simulink model "supervisoryController_ref"  (R2019b)
settings: Solver=FixedStepDiscrete  StartTime=0.0  StopTime=10  FixedStep=0.01  RelTol=1e-3  EnableMultiTasking=on
PreLoadFcn:
  | Ts1 = 0.01;
  | Ts2 = 0.1;
InitFcn:
  | initACCParams_pid;
model workspace (MAT data in the model file):
  firstWarning = 1
  originalScenarioChecksum = '3C3E23DDE530CB8BEC76DD6DBB66960A'
undefined symbols (not defined in the file): default_spacing, DiscIntNeverNeededParam, time_gap
libraries: simulink x1
settings Model: EnablePacing=on  Creator=sseshadr  LastModifiedBy=cdsouza
settings SolverCC: AutoInsertRateTranBlk=on
settings DataIOCC: SaveOutput=off  SaveTime=off
settings OptimizationCC: GainParamInheritBuiltInType=on  UseFloatMulNetSlope=on  EnableMemcpy=off  PassReuseOutputArgsAs=Individual arguments  ZeroExternalMemoryAtStartup=off  ZeroInternalMemoryAtStartup=off  NoFixptDivByZeroProtection=on  EfficientFloat2IntCast=on  LifeSpan=1  OptimizeBlockOrder=speed  DifferentSizesBufferReuse=on  EfficientTunableParamExpr=on
settings DebuggingCC: ParameterTunabilityLossMsg=error
settings HardwareCC: ProdLongLongMode=on
settings SFSimCC: MATLABDynamicMemAlloc=off
settings RTWCC: SystemTargetFile=ert.tlc  TemplateMakefile=ert_default_tmf  GenerateReport=on  IncludeHyperlinkInReport=on  LaunchReport=on  GenerateTraceInfo=on  GenerateTraceReport=on  GenerateTraceReportSl=on  GenerateTraceReportSf=on  GenerateTraceReportEml=on  GenerateCodeMetricsReport=on
settings CodeAppCC: ForceParamTrailComments=on  IgnoreCustomStorageClasses=off  OperatorAnnotations=on  SimulinkDataObjDesc=on  SFDataObjDesc=on  CustomSymbolStrGlobalVar=rt$N$M  CustomSymbolStrType=$N$M  CustomSymbolStrFcn=$N$M$F  CustomSymbolStrMacro=$N$M  InsertBlockDesc=on
settings ERTTargetCC: TargetLangStandard=C99 (ISO)  GenerateSampleERTMain=on  IncludeMdlTerminateFcn=off  CombineSignalStateStructs=on  SupportAbsoluteTime=off  SupportComplex=off  SupportNonInlinedSFcns=on  ERTCustomFileTemplate=example_file_process.tlc

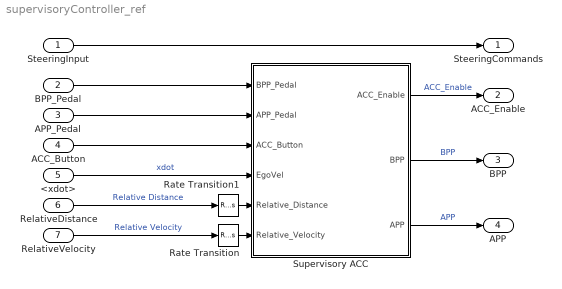
== system supervisoryController_ref ==
  "SteeringInput " : Inport  OutDataTypeStr=double  PortDimensions=1  SampleTime=Ts1
  BPP_Pedal : Inport  Port=2  OutDataTypeStr=double  PortDimensions=1  SampleTime=Ts1
  APP_Pedal : Inport  Port=3  OutDataTypeStr=double  PortDimensions=1  SampleTime=Ts1
  ACC_Button : Inport  Port=4  OutDataTypeStr=double  PortDimensions=1  SampleTime=Ts1
  <xdot> : Inport  Port=5  OutDataTypeStr=double  PortDimensions=1  SampleTime=Ts1
  RelativeDistance : Inport  Port=6  OutDataTypeStr=double  PortDimensions=[1 1]  SampleTime=Ts2
  RelativeVelocity : Inport  Port=7  OutDataTypeStr=double  PortDimensions=[1 1]  SampleTime=Ts2
  Rate Transition : RateTransition
  Rate Transition1 : RateTransition
  Supervisory ACC : Stateflow chart  BlockKeywords=__PRM__SERIALIZED__DATA__:Stateflow Chart,Stateflow Diagram  TreatAsAtomicUnit=on
  SteeringCommands : Outport  OutDataTypeStr=double  PortDimensions=1
  ACC_Enable : Outport  Port=2  OutDataTypeStr=double  PortDimensions=1
  BPP : Outport  Port=3  OutDataTypeStr=double  PortDimensions=1
  APP : Outport  Port=4  OutDataTypeStr=double  PortDimensions=1
  wires:
  BPP_Pedal/1 -> Supervisory ACC/1(BPP_Pedal)
  Supervisory ACC/2(BPP) -> BPP/1  "BPP"
  Supervisory ACC/3(APP) -> APP/1  "APP"
  Supervisory ACC/1(ACC_Enable) -> ACC_Enable/1  "ACC_Enable"
  RelativeDistance/1 -> Rate Transition1/1  "Relative Distance"
  ACC_Button/1 -> Supervisory ACC/3(ACC_Button)
  <xdot>/1 -> Supervisory ACC/4(EgoVel)  "xdot"
  APP_Pedal/1 -> Supervisory ACC/2(APP_Pedal)
  "SteeringInput "/1 -> SteeringCommands/1
  RelativeVelocity/1 -> Rate Transition/1  "Relative Velocity"
  Rate Transition/1 -> Supervisory ACC/6(Relative_Velocity)
  Rate Transition1/1 -> Supervisory ACC/5(Relative_Distance)

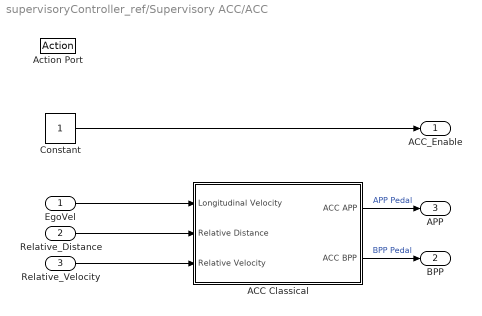
== system supervisoryController_ref/Supervisory ACC/ACC ==
  EgoVel : Inport
  Relative_Distance : Inport  Port=2
  Relative_Velocity : Inport  Port=3
  Action Port : ActionPort
      settings: CopyFcn=Stateflow.SLINSF.SimulinkMan.removeBlockPreDeleteFcn  PreDeleteFcn=Stateflow.SLINSF.SimulinkMan.unsafePredeleteFcn
  ACC Classical : Subsystem  VariantControl=controller_type == 1
      settings: RTWFileNameOpts=Use function name
  Constant : Constant  SampleTime=-1
  ACC_Enable : Outport
  BPP : Outport  Port=2
  APP : Outport  Port=3
  wires:
  Constant/1 -> ACC_Enable/1
  ACC Classical/2(ACC BPP) -> BPP/1  "BPP Pedal"
  ACC Classical/1(ACC APP) -> APP/1  "APP Pedal"
  Relative_Velocity/1 -> ACC Classical/3(Relative Velocity)
  Relative_Distance/1 -> ACC Classical/2(Relative Distance)
  EgoVel/1 -> ACC Classical/1(Longitudinal Velocity)

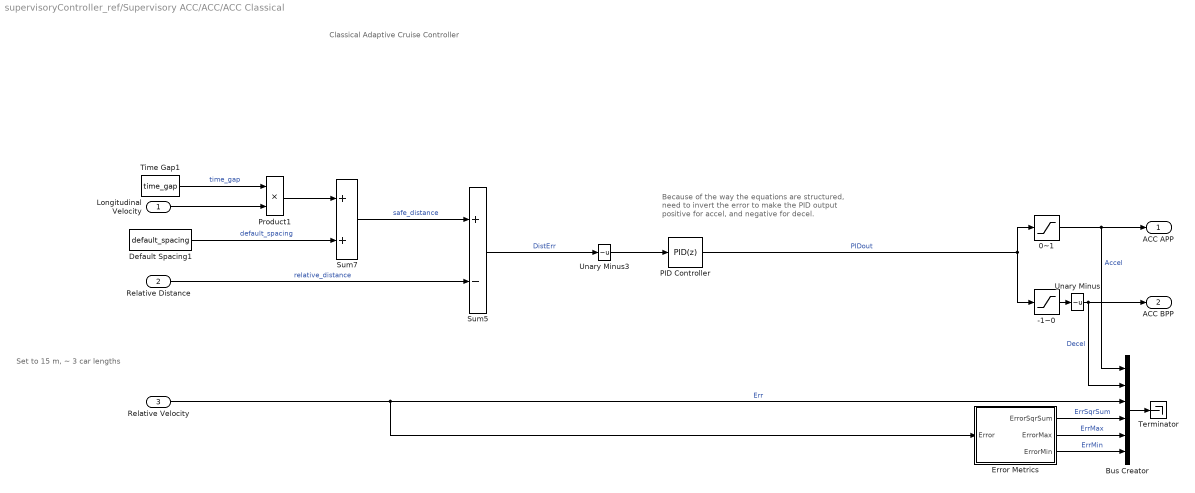
== system supervisoryController_ref/Supervisory ACC/ACC/ACC Classical ==
  note: Classical Adaptive Cruise Controller
  note: Set to 15 m, ~ 3 car lengths
  note: Because of the way the equations are structured,
      | need to invert the error to make the PID output
      | positive for accel, and negative for decel.
  Longitudinal Velocity : Inport
  Relative Distance : Inport  Port=2
  Relative Velocity : Inport  Port=3
  -1~0 : Saturate  UpperLimit=0  LowerLimit=-1  ZeroCross=off
  0~1 : Saturate  UpperLimit=1  LowerLimit=0  ZeroCross=off
  Bus Creator : BusCreator  Inputs=6
  Default Spacing1 : Constant  Value=default_spacing  SampleTime=-1
  Error Metrics : Subsystem
  PID Controller : simulink/Continuous/PID Controller  Controller=PID  Form=Parallel  TimeDomain=Discrete-time  SampleTime=-1  IntegratorMethod=Forward Euler  FilterMethod=Forward Euler  ControllerParametersSource=internal  P=0.05  I=0.001  D=0.05  UseFilter=on  N=10  TunerSelectOption=Transfer Function Based (PID Tuner App)  InitialConditionSource=internal  InitialConditionForIntegrator=0  InitialConditionForFilter=0  DifferentiatorICPrevScaledInput=0  ExternalReset=none  TrackingMode=off  Kt=1  LimitOutput=on  UpperSaturationLimit=1  LowerSaturationLimit=-1  LinearizeAsGain=on  AntiWindupMode=clamping  Kb=1  POutMin=[]  POutMax=[]  IOutMin=[]  IOutMax=[]  DOutMin=[]  DOutMax=[]  NOutMin=[]  NOutMax=[]  SumOutMin=[]  SumOutMax=[]  SaturationOutMin=[]  SaturationOutMax=[]  PParamMin=[]  PParamMax=[]  IParamMin=[]  IParamMax=[]  DParamMin=[]  DParamMax=[]  NParamMin=[]  NParamMax=[]  KbParamMin=[]  KbParamMax=[]  KtParamMin=[]  KtParamMax=[]  KbOutMin=[]  KbOutMax=[]  KtOutMin=[]  KtOutMax=[]  IntegratorOutMin=[]  IntegratorOutMax=[]  FilterOutMin=[]  FilterOutMax=[]  SumI1OutMin=[]  SumI1OutMax=[]  SumI2OutMin=[]  SumI2OutMax=[]  SumI3OutMin=[]  SumI3OutMax=[]  SumI4OutMin=[]  SumI4OutMax=[]  SumDOutMin=[]  SumDOutMax=[]  DifferentiatorOutMin=[]  DifferentiatorOutMax=[]  FilterDiffOutCoefMin=[]  FilterDiffOutCoefMax=[]  ReciprocalOutMin=[]  ReciprocalOutMax=[]  SumDenOutMin=[]  SumDenOutMax=[]  SumNumOutMin=[]  SumNumOutMax=[]  DivideOutMin=[]  DivideOutMax=[]  IntegratorContinuousStateAttributes=''  IntegratorStateMustResolveToSignalObject=off  IntegratorRTWStateStorageClass=Auto  FilterContinuousStateAttributes=''  FilterStateMustResolveToSignalObject=off  FilterRTWStateStorageClass=Auto  ParallelPVariant=InternalParameters  IdealPVariant=Disabled  IVariant=InternalParameters  DVariant=InternalParameters  IntegratorVariant=Discrete  SatVariant=Enabled  AWVariant=DiscClampingParallel  PCopyVariant=Disabled  TRVariant=Disabled  FdbkBlocksVariant=Forward  IdealPFdbkVariant=Disabled  SatFdbkVariant=Disabled  DerivativeFilterVariant=ForwardEulerFilter  NVariant=InternalParameters  NCopyVariant=Disabled  FilterICVariant=InternalICsFilter  IntegratorICVariant=InternalICs  ExternalResetVariant=Disabled  TRSumVariant=Passthrough  SumFdbkVariant=Disabled  SumVariant=Sum_PID
  Product1 : Product
  Sum5 : Sum  Inputs=+-
  Sum7 : Sum
  Terminator : Terminator
  Time Gap1 : Constant  Value=time_gap  SampleTime=-1
  Unary Minus : UnaryMinus
  Unary Minus3 : UnaryMinus
  ACC APP : Outport  Unit=one  InitialOutput=0  VectorParamsAs1DForOutWhenUnconnected=off
  ACC BPP : Outport  Port=2  Unit=one  InitialOutput=0  VectorParamsAs1DForOutWhenUnconnected=off
  wires:
  Error Metrics/2(ErrorMax) -> Bus Creator/5  "ErrMax"
  Default Spacing1/1 -> Sum7/2  "default_spacing"
  Sum7/1 -> Sum5/1  "safe_distance"
  Sum5/1 -> Unary Minus3/1  "DistErr"
  Unary Minus/1 -> Bus Creator/2, ACC BPP/1  "Decel"
  Product1/1 -> Sum7/1
  Relative Distance/1 -> Sum5/2  "relative_distance"
  Longitudinal Velocity/1 -> Product1/2
  Bus Creator/1 -> Terminator/1
  0~1/1 -> ACC APP/1, Bus Creator/1  "Accel"
  Time Gap1/1 -> Product1/1  "time_gap"
  Error Metrics/1(ErrorSqrSum) -> Bus Creator/4  "ErrSqrSum"
  -1~0/1 -> Unary Minus/1
  PID Controller/1 -> -1~0/1, 0~1/1  "PIDout"
  Unary Minus3/1 -> PID Controller/1
  Relative Velocity/1 -> Bus Creator/3, Error Metrics/1(Error)  "Err"
  Error Metrics/3(ErrorMin) -> Bus Creator/6  "ErrMin"

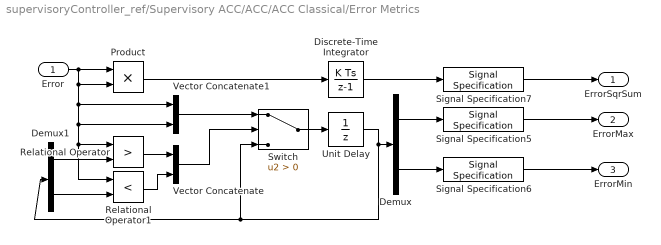
== system supervisoryController_ref/Supervisory ACC/ACC/ACC Classical/Error Metrics ==
  Error : Inport
  Demux : Demux  Outputs=2
  Demux1 : Demux  Outputs=2
  Discrete-Time Integrator : DiscreteIntegrator  SampleTime=-1  ICPrevOutput=DiscIntNeverNeededParam  ICPrevScaledInput=DiscIntNeverNeededParam
  Product : Product
  Relational Operator : RelationalOperator  Operator=>  OutDataTypeStr=boolean  ZeroCross=off  RndMeth=Simplest
  Relational Operator1 : RelationalOperator  Operator=<  OutDataTypeStr=boolean  ZeroCross=off  RndMeth=Simplest
  Signal Specification5 : SignalSpecification  Unit=m/s
  Signal Specification6 : SignalSpecification  Unit=m/s
  Signal Specification7 : SignalSpecification  Unit=m^2/s^2
  Switch : Switch  Criteria=u2 > Threshold
  Unit Delay : UnitDelay  InitialCondition=[0,0]  SampleTime=-1  HasFrameUpgradeWarning=on
  Vector Concatenate : Concatenate
  Vector Concatenate1 : Concatenate
  ErrorSqrSum : Outport  VectorParamsAs1DForOutWhenUnconnected=off
  ErrorMax : Outport  Port=2  VectorParamsAs1DForOutWhenUnconnected=off
  ErrorMin : Outport  Port=3  VectorParamsAs1DForOutWhenUnconnected=off
  wires:
  Discrete-Time Integrator/1 -> Signal Specification7/1
  Product/1 -> Discrete-Time Integrator/1
  Error/1 -> Product/2, Vector Concatenate1/2, Relational Operator1/1, Relational Operator/1, Vector Concatenate1/1, Product/1
  Switch/1 -> Unit Delay/1
  Unit Delay/1 -> Switch/3, Demux1/1, Demux/1
  Relational Operator1/1 -> Vector Concatenate/2
  Relational Operator/1 -> Vector Concatenate/1
  Vector Concatenate1/1 -> Switch/1
  Demux/1 -> Signal Specification5/1
  Demux/2 -> Signal Specification6/1
  Demux1/2 -> Relational Operator1/2
  Demux1/1 -> Relational Operator/2
  Vector Concatenate/1 -> Switch/2
  Signal Specification7/1 -> ErrorSqrSum/1
  Signal Specification6/1 -> ErrorMin/1
  Signal Specification5/1 -> ErrorMax/1

== stateflow chart supervisoryController_ref/Supervisory ACC ==
  state WaitOff
  state Normal
    during:
    APP = APP_Pedal;
    BPP = BPP_Pedal;
    ACC_Enable = 0;
  state ACC
  state WaitOn
  WaitOff -> Normal : [ACC_Button == -1]
  ACC -> WaitOff [order 2] : [ACC_Button == 180]
  (default) -> Normal
  ACC -> Normal [order 1] : [APP_Pedal || BPP_Pedal > 0]
  WaitOn -> ACC : [ACC_Button == -1]
  Normal -> WaitOn : [ACC_Button == 180]
  data: sf_internal_action_state_placeholder_data local double size=1 =0; ACC_Enable output; BPP output; APP output; BPP_Pedal input; APP_Pedal input; ACC_Button input; EgoVel input; Relative_Distance input; Relative_Velocity input
